simulink model "mass_sim"  (R2015a)
settings: Solver=ode45  StartTime=0.0  StopTime=100  RelTol=1e-3
InitFcn:
  | param
undefined symbols (not defined in the file or in its folder): drawMSD, P
settings Model: Creator=beard  LastModifiedBy=beard
settings DataIOCC: SignalLoggingSaveFormat=ModelDataLogs
settings OptimizationCC: ExpressionDepthLimit=2147483647  InitFltsAndDblsToZero=on
settings DebuggingCC: UnderspecifiedInitializationDetection=Classic  MergeDetectMultiDrivingBlocksExec=none  SolverPrmCheckMsg=warning  FcnCallInpInsideContextMsg=UseLocalSettings  StateNameClashWarn=warning
settings GRTTargetCC: CombineOutputUpdateFcns=off  GRTInterface=on

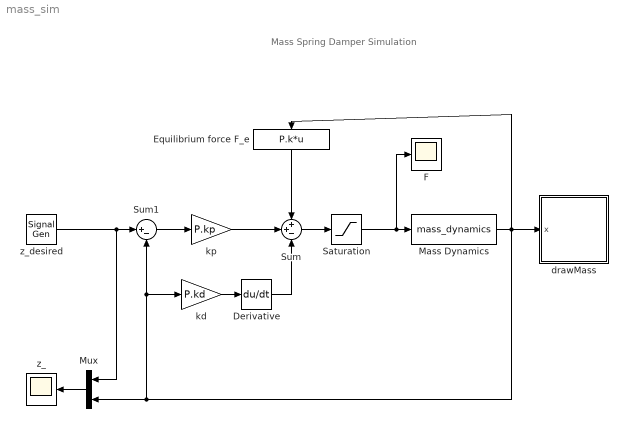
== system mass_sim ==
  note: Mass Spring Damper Simulation
  Derivative : Derivative
  Equilibrium force F_e : Fcn  Expr=P.k*u
  F : Scope
      settings: TimeRange=100  YMin=-1.75  YMax=2
  Mass Dynamics : S-Function  FunctionName=mass_dynamics  Parameters=AP
  Mux : Mux  Inputs=2
  Saturation : Saturate  UpperLimit=P.Fmax  LowerLimit=-P.Fmax
  Sum : Sum  Inputs=++-
  Sum1 : Sum  Inputs=|+-
  drawMass : Subsystem
      mask Display: image(imread('tv.jpg'))
  kd : Gain  Gain=P.kd
  kp : Gain  Gain=P.kp
  z_ : Scope
      settings: TimeRange=100  YMin=-2  YMax=1.5
  z_desired : SignalGenerator  WaveForm=square  Amplitude=.5  Frequency=.02
  wires:
  Sum/1 -> Saturation/1
  Sum1/1 -> kp/1
  z_desired/1 -> Sum1/1, Mux/1
  Mass Dynamics/1 -> Equilibrium force F_e/1, kd/1, Sum1/2, Mux/2, drawMass/1(x)
  Mux/1 -> z_/1
  kp/1 -> Sum/2
  kd/1 -> Derivative/1
  Derivative/1 -> Sum/3
  Saturation/1 -> F/1, Mass Dynamics/1
  Equilibrium force F_e/1 -> Sum/1

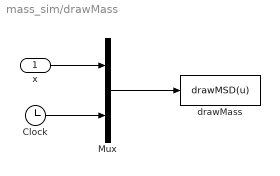
== system mass_sim/drawMass ==
  x : Inport
  Clock : Clock
  Mux : Mux  Inputs=2
  drawMass : MATLABFcn  MATLABFcn=drawMSD(u)  OutputDimensions=0  SampleTime=0.1
  wires:
  Clock/1 -> Mux/2
  x/1 -> Mux/1
  Mux/1 -> drawMass/1
